simulink model "Ejercicio4_simulink"  (R2016a)
settings: Solver=VariableStepAuto  StartTime=0.0  StopTime=800  RelTol=1e-3
settings Model: Creator=estebanza  LastModifiedBy=estebanza

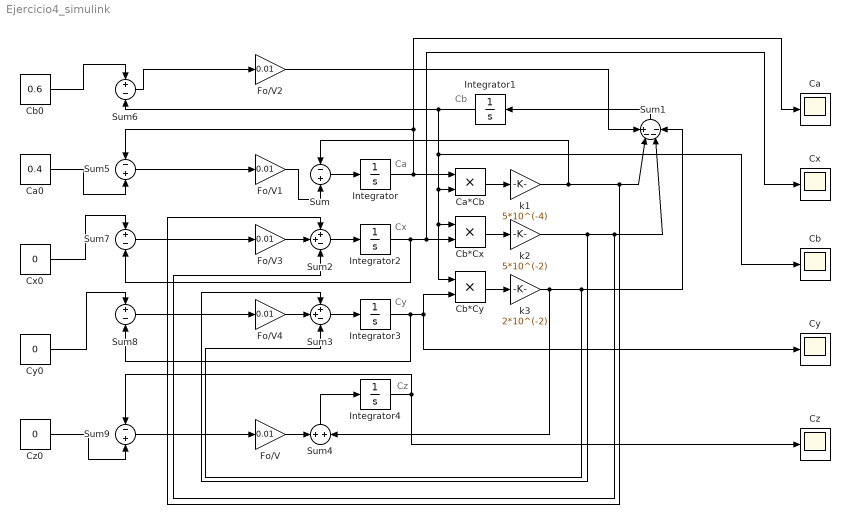
== system Ejercicio4_simulink ==
  note: Cx
  note: Cb
  note: Ca
  note: Cy
  note: Cz
  Ca : Scope
  Ca*Cb : Product
  Ca0 : Constant  Value=0.4
  Cb : Scope
  Cb*Cx : Product
  Cb*Cy : Product
  Cb0 : Constant  Value=0.6
  Cx : Scope
  Cx0 : Constant  Value=0
  Cy : Scope
  Cy0 : Constant  Value=0
  Cz : Scope
  "Cz0 " : Constant  Value=0
  Fo/V{,1..4} (5 alike) : Gain  Gain=0.01
  Integrator{,1..4} (5 alike) : Integrator
  Sum : Sum  Inputs=-+
  Sum1 : Sum  Inputs=+---
  Sum2 : Sum  Inputs=++-
  Sum3 : Sum  Inputs=++-
  Sum4 : Sum
  Sum5 : Sum  Inputs=-+
  Sum6 : Sum  Inputs=+-
  Sum7 : Sum  Inputs=+-
  Sum8 : Sum  Inputs=+-
  Sum9 : Sum  Inputs=-+
  k1 : Gain  Gain=5*10^(-4)
  k2 : Gain  Gain=5*10^(-2)
  k3 : Gain  Gain=2*10^(-2)
  wires:
  Sum/1 -> Integrator/1
  k1/1 -> Sum2/1, Sum1/2, Sum/1
  k2/1 -> Sum2/3, Sum1/3, Sum3/1
  k3/1 -> Sum4/2, Sum1/4, Sum3/3
  Sum1/1 -> Integrator1/1
  Cb*Cx/1 -> k2/1
  Cb*Cy/1 -> k3/1
  Integrator2/1 -> Cb*Cx/2, Cx/1, Sum7/2
  Sum2/1 -> Integrator2/1
  Ca*Cb/1 -> k1/1
  Fo/V2/1 -> Sum1/1
  Fo/V3/1 -> Sum2/2
  Integrator3/1 -> Cb*Cy/2, Cy/1, Sum8/2
  Sum3/1 -> Integrator3/1
  Sum4/1 -> Integrator4/1
  Cb0/1 -> Sum6/1
  Cx0/1 -> Sum7/1
  Cy0/1 -> Sum8/1
  "Cz0 "/1 -> Sum9/2
  Integrator4/1 -> Cz/1, Sum9/1
  Sum9/1 -> Fo/V/1
  Fo/V/1 -> Sum4/1
  Sum5/1 -> Fo/V1/1
  Fo/V1/1 -> Sum/2
  Ca0/1 -> Sum5/2
  Integrator/1 -> Sum5/1, Ca/1, Ca*Cb/1
  Integrator1/1 -> Cb*Cy/1, Cb*Cx/1, Ca*Cb/2, Cb/1, Sum6/2
  Sum6/1 -> Fo/V2/1
  Sum7/1 -> Fo/V3/1
  Fo/V4/1 -> Sum3/2
  Sum8/1 -> Fo/V4/1
